simulink model "EstimateOrientationUsingAHRSandIMU"  (R2023a)
settings: Solver=FixedStepAuto  StartTime=0.0  StopTime=inf  RelTol=1e-3  EnableMultiTasking=on
libraries: arduinosensorlib x2, mspfiltlib x1
settings Model: ExtModeTrigDuration=2  Creator=The MathWorks, Inc.  LastModifiedBy=Clément
settings SolverCC: MaxZcPerStep=1
settings OptimizationCC: EnhancedBackFolding=on  PassReuseOutputArgsThreshold=0  MaxStackSize=64  OptimizeBlockOrder=speed  DifferentSizesBufferReuse=on  OptimizationCustomize=off
settings DebuggingCC: ParameterPrecisionLossMsg=none  ParameterTunabilityLossMsg=error  UnconnectedInputMsg=warning  UnconnectedOutputMsg=warning  UnconnectedLineMsg=warning
settings HardwareCC: ProdBitPerPointer=32  ProdBitPerSizeT=32  ProdBitPerPtrDiffT=32  ProdLargestAtomicInteger=Long  ProdLargestAtomicFloat=Double  ProdWordSize=32  ProdHWDeviceType=ARM Compatible->ARM Cortex  UseEmbeddedCoderFeatures=off
settings ModelReferenceCC: EnableRefExpFcnMdlSchedulingChecks=on
settings SFSimCC: MATLABDynamicMemAlloc=off
settings RTWCC: Description=Embedded Coder  SystemTargetFile=ert.tlc  HardwareBoard=Arduino MKR1000  TemplateMakefile=ert_default_tmf  Toolchain=Arduino ARM  BuildConfiguration=Faster Runs  DLArmComputeVersion=19.05
settings CodeAppCC: ForceParamTrailComments=on  OperatorAnnotations=on
settings ERTTargetCC: ERTCustomFileBanners=off  SupportContinuousTime=on  SupportNonInlinedSFcns=on  RemoveResetFunc=off  SupportVariableSizeSignals=on  ModelStepFunctionPrototypeControlCompliant=off  ExtModeTransport=3  ExtModeStaticAlloc=on  ExtModeAutomaticAllocSize=off  ExtModeStaticAllocSize=8192  ExtModeMexFile=ext_xcp  ExtModeIntrfLevel=Level2 - Open

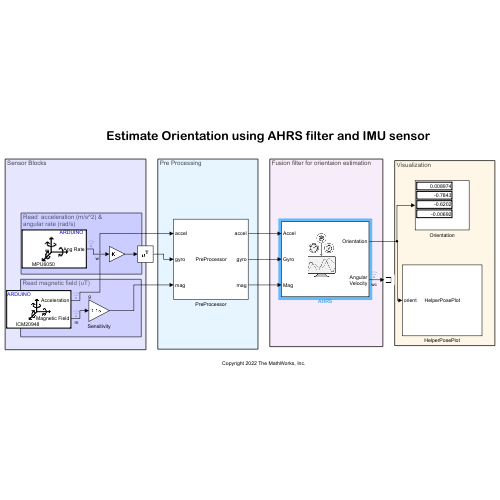
[thumbnail: Simulink's stored preview of the top-level diagram]
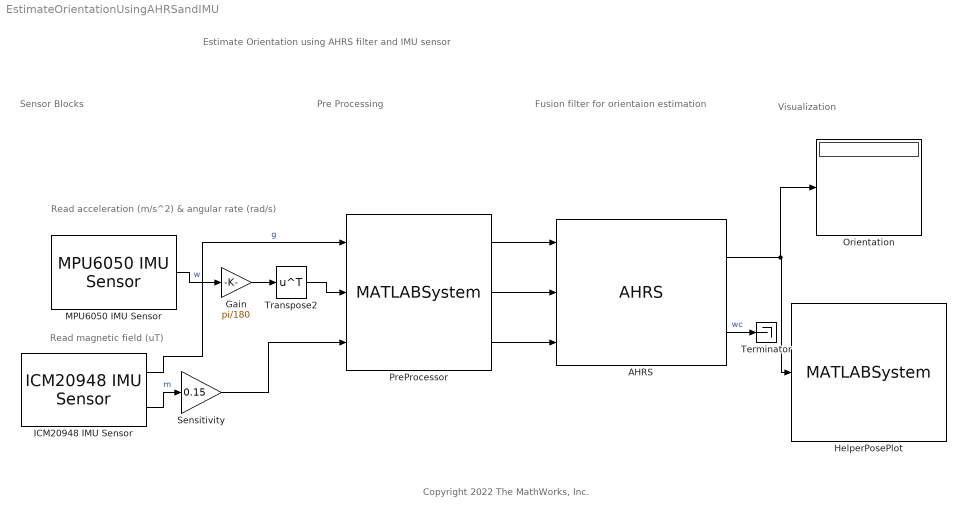
== system EstimateOrientationUsingAHRSandIMU ==
  note: Visualization
  note: Fusion filter for orientaion estimation
  note: Pre Processing
  note: Read  acceleration (m/s^2) &
      | angular rate (rad/s)
  note: Read magnetic field (uT)
  note: Sensor Blocks
  note: Copyright 2022 The MathWorks, Inc.
  note: Estimate Orientation using AHRS filter and IMU sensor
  AHRS : mspfiltlib/AHRS  DispRefFrame=ENU  DecimationFactor=1  InitialProcessNoise=ahrsfilter.defaultProcessNoise  OrientationFormat=quaternion  SimulateUsing=Interpreted execution  AccelerometerNoise=0.0001924722  GyroscopeNoise=9.1385e-5  MagnetometerNoise=0.1  GyroscopeDriftNoise=12.0462e-13  LinearAccelerationNoise=0.0096236100000000012  MagneticDisturbanceNoise=0.5  LinearAccelerationDecayFactor=0.5  MagneticDisturbanceDecayFactor=0.5  ExpectedMagneticFieldStrength=50
  Gain : Gain  Gain=pi/180
  HelperPosePlot : MATLABSystem  System=HelperPosePlot  OrientationFormat=Quaternion
      mask Type: HelperPosePlot
      mask Display:
      | disp('HelperPosePlot');
      | port_label('input',1,'orient');
  ICM20948 IMU Sensor : arduinosensorlib/ICM20948 IMU Sensor  I2CAddress=0x69  BitRate=1000000  EnableDRDY=off  InterruptType=Active high  IsActiveAccel=on  IsActiveGyro=off  IsActiveMag=on  IsActiveTemp=off  IsActiveStatus=off  IsActiveTimeStamp=off  AccelerometerRange=+/-2g  AccelerometerODR=1125  AccelerometerBW=23.9 Hz  GyroscopeRange=+/-250 dps  GyroscopeODR=1125  GyroscopeBW=23.9 Hz  MagnetometerODR=100 Hz  TemperatureBW=34.1 Hz  DataType=double  spf=1  SampleTime=-1  QueueSizeFactor=1
  MPU6050 IMU Sensor : arduinosensorlib/MPU6050 IMU Sensor  SlaveAddress=0x68  Accel=off  AngularRate=on  Temperature=off  Status=off  Timestamp=off  EulerAngles=off  Quat=off  AccelRange=2G  GyroRange=250 dps  DmpOdr=200 Hz  Dlpf=Accelerometer: 184Hz, Gyroscope: 188Hz  spf=1  SampleTime=-1  QueueSizeFactor=1
  Orientation : Display
  PreProcessor : MATLABSystem  System=PreProcessor  MagOffsets=[-3.7477,2.6230,9.3852]  AccelXAxisIndex=2  AccelXAxisSign=-  AccelYAxisIndex=1  AccelYAxisSign=-  AccelZAxisIndex=3  AccelZAxisSign=-  GyroXAxisIndex=2  GyroXAxisSign=+  GyroYAxisIndex=1  GyroYAxisSign=-  GyroZAxisIndex=3  GyroZAxisSign=+  MagXAxisIndex=2  MagXAxisSign=-  MagYAxisIndex=1  MagYAxisSign=-  MagZAxisIndex=3  MagZAxisSign=-
      mask Type: PreProcessor
      mask Display:
      | disp('PreProcessor');
      | port_label('input',1,'accel');
      | port_label('input',2,'gyro');
      | port_label('input',3,'mag');
      | port_label('output',1,'accel');
      | port_label('output',2,'gyro');
      | port_label('output',3,'mag');
  Sensitivity : Gain  Gain=0.15  OutDataTypeStr=double  LockScale=on
  Terminator : Terminator
  Transpose2 : Math  Operator=transpose
  wires:
  ICM20948 IMU Sensor/2 -> Sensitivity/1  "m"
  ICM20948 IMU Sensor/1 -> PreProcessor/1  "g"
  MPU6050 IMU Sensor/1 -> Gain/1  "w"
  Sensitivity/1 -> PreProcessor/3
  PreProcessor/2 -> AHRS/2
  AHRS/2 -> Terminator/1  "wc"
  PreProcessor/1 -> AHRS/1
  PreProcessor/3 -> AHRS/3
  AHRS/1 -> Orientation/1, HelperPosePlot/1
  Transpose2/1 -> PreProcessor/2
  Gain/1 -> Transpose2/1
